simulink model "test_autopilot"  (R2015b)
settings: Solver=ode45  StartTime=0.0  StopTime=10  RelTol=1e-3
undefined symbols (not defined in the file or in its folder): sigbuilder_block
settings Model: Creator=rcasado  LastModifiedBy=rcasado
settings DataIOCC: SaveFormat=Array
settings DebuggingCC: UnderspecifiedInitializationDetection=Classic  MergeDetectMultiDrivingBlocksExec=none  SolverPrmCheckMsg=warning  MultiTaskDSMMsg=warning  MultiTaskCondExecSysMsg=none  StateNameClashWarn=warning  StrictBusMsg=None
settings HardwareCC: ProdBitPerPointer=32  ProdLargestAtomicFloat=None  ProdIntDivRoundTo=Undefined  ProdEndianess=Unspecified  ProdWordSize=32  ProdHWDeviceType=32-bit Generic
settings GRTTargetCC: GeneratePreprocessorConditionals=Disable all
settings ConfigComp: CovModelRefEnable=Off

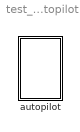
== system test_autopilot ==
  autopilot : Subsystem

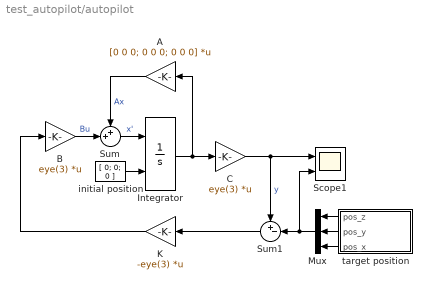
== system test_autopilot/autopilot ==
  A : Gain  Gain=[0 0 0; 0 0 0; 0 0 0]  Multiplication=Matrix(K*u)
  B : Gain  Gain=eye(3)  Multiplication=Matrix(K*u)
  C : Gain  Gain=eye(3)  Multiplication=Matrix(K*u)
  Integrator : Integrator  InitialConditionSource=external  InitialCondition=[3; 1]
  K : Gain  Gain=-eye(3)  Multiplication=Matrix(K*u)
  Mux : Mux  Inputs=3
  Scope1 : Scope  NumInputPorts=2
  Sum : Sum  Inputs=++|
  Sum1 : Sum  Inputs=+-|
  initial position : Constant  Value=[ 0; 0; 0 ]
  target position : Subsystem  Tag=STV Subsys  LoadFcn=sigbuilder_block('load');  StartFcn=sigbuilder_block('start');  StopFcn=sigbuilder_block('stop');  ClipboardFcn=sigbuilder_block('clipboard');  mask(Sigbuilder block){}
      mask help: Simulink:masks:SigbuilderBlock_MD
      mask init:
      | if ~strcmp(get_param(bdroot(gcbh),'SimulationStatus'),'stopped') tuvar = sigbuilder_block('maskInit'); end
      settings: CopyFcn=sigbuilder_block('copy');  DeleteFcn=sigbuilder_block('delete');  ModelCloseFcn=sigbuilder_block('modelClose');  PreSaveFcn=sigbuilder_block('preSave');  PauseFcn=sigbuilder_block('pause');  ContinueFcn=sigbuilder_block('continue');  NameChangeFcn=sigbuilder_block('namechange');  OpenFcn=sigbuilder_block('open',[402 166.2 550.8 400.2 ]);  CloseFcn=sigbuilder_block('close');
      mask Display: plot(0, 0, 100, 100,[2, 2, 32, 32, 2], [68, 8, 8, 68, 68],[32, 2], [38, 38], [32, 19, 2],[53, 60, 44], [32, 17, 17, 2],[16, 16, 31, 31]);txt = getActiveGroup(gcbh);text(2, 100, txt,'verticalAlignment', 'top');
  wires:
  C/1 -> Sum1/1, Scope1/1  "y"
  target position/1(pos_z) -> Mux/1
  Mux/1 -> Scope1/2, Sum1/2
  target position/3(pos_x) -> Mux/3
  target position/2(pos_y) -> Mux/2
  A/1 -> Sum/1  "Ax"
  B/1 -> Sum/2  "Bu"
  Integrator/1 -> A/1, C/1
  Sum/1 -> Integrator/1  "x'"
  initial position/1 -> Integrator/2
  K/1 -> B/1
  Sum1/1 -> K/1

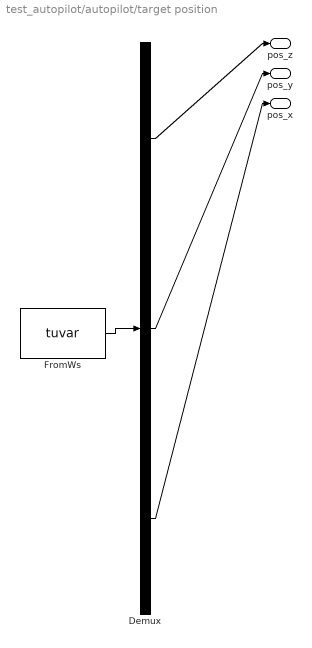
== system test_autopilot/autopilot/target position ==
  Demux : Demux  Tag=STV Demux  Outputs=3
  FromWs : FromWorkspace  Tag=STV FromWs  VariableName=tuvar  SampleTime=0
      SigBuilderData=|
      | common.afterFinalStr = 'Extrapolate'
      | common.sampleTime = 0
      | dataSet.timeRange = [0 10]
      | dataSet.name = 'Group 1'
      | sbobj.Groups.Name = 'Group 1'
      | sbobj.Groups.Signals(1).Name = 'pos_z'
      | sbobj.Groups.Signals(1).XData = [0 10]
      | sbobj.Groups.Signals(1).YData = [0 0]
      | sbobj.Groups.Signals(2).Name = 'pos_y'
      | sbobj.Groups.Signals(2).XData = [0 10]
      | sbobj.Groups.Signals(2).YData = [0 0]
      | sbobj.Groups.Signals(3).Name = 'pos_x'
      | sbobj.Groups.Signals(3).XData = [0 2 2 4 6 10]
      | sbobj.Groups.Signals(3).YData = [0 0 3 3 3 3]
  pos_z : Outport  Tag=STV Outport
  pos_y : Outport  Tag=STV Outport  Port=2
  pos_x : Outport  Tag=STV Outport  Port=3
  wires:
  FromWs/1 -> Demux/1
  Demux/1 -> pos_z/1
  Demux/2 -> pos_y/1
  Demux/3 -> pos_x/1
